simulink model "NMPC_sim"  (R2024b)
settings: Solver=ode4  StartTime=0.0  StopTime=inf  FixedStep=1/60  RelTol=1e-3
values from neighbouring files (symbols this model uses):
  alpha = 2.5    [pre_nmpc_simulink.m]    (also in pre_nmpc_simulink_d10.m = 6.3; pre_nmpc_simulink_d11.m = 7.3; pre_nmpc_simulink_d12.m = 5.8; pre_nmpc_simulink_d13.m = 5.8)
  d = 0.5    [NMPC_System.m]    (also in pre_nmpc_simulink.m = 0.393; pre_nmpc_simulink_d10.m = 0.393; pre_nmpc_simulink_d11.m = 0.393; pre_nmpc_simulink_d12.m = 0.393)
  eta = 0.7    [pre_nmpc_simulink.m]    (also in pre_nmpc_simulink_d10.m = 1.9; pre_nmpc_simulink_d11.m = 1.9; pre_nmpc_simulink_d12.m = 1.4; pre_nmpc_simulink_d13.m = 1.5)
  N = 20    [NMPC_System.m]    (also in pre_nmpc_simulink.m; pre_nmpc_simulink_d10.m; pre_nmpc_simulink_d11.m; pre_nmpc_simulink_d12.m)
  Q_cost = diag([1, 1, 0.1])    [NMPC_System.m]    (also in pre_nmpc_simulink.m = diag([100, 100, 10]); pre_nmpc_simulink_d10.m = diag([100, 100, 10]); pre_nmpc_simulink_d11.m = diag([100, 100, 10]); pre_nmpc_simulink_d12.m = diag([100, 100, 10]))
  r = 0.1    [NMPC_System.m]    (also in pre_nmpc_simulink.m = 0.04445; pre_nmpc_simulink_d10.m = 0.04445; pre_nmpc_simulink_d11.m = 0.04445; pre_nmpc_simulink_d12.m = 0.04445)
  R_cost = diag([0.01, 0.01])    [NMPC_System.m]    (also in pre_nmpc_simulink.m = diag([0.2, 0.1]); pre_nmpc_simulink_d10.m = diag([1.7, 0.1]); pre_nmpc_simulink_d11.m = diag([1.7, 0.1]); pre_nmpc_simulink_d12.m = diag([1.7, 0.1]))
  ts = 0.1    [NMPC_System.m]    (also in pre_nmpc_simulink.m = 0.0166666666667; pre_nmpc_simulink_d10.m = 0.0166666666667; pre_nmpc_simulink_d11.m = 0.0166666666667; pre_nmpc_simulink_d12.m = 0.0166666666667)
  wrwlmax = 10.0    (= 10)    [pre_nmpc_simulink.m]    (also in pre_nmpc_simulink_d10.m; pre_nmpc_simulink_d11.m; pre_nmpc_simulink_d12.m; pre_nmpc_simulink_d13.m)
libraries: simulink x4, quarc_library x3
settings Model: PacingRate=0.032000  Creator=umroot  LastModifiedBy=umroot

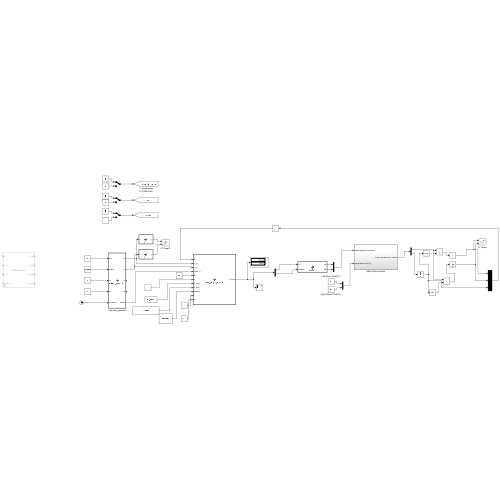
[thumbnail: Simulink's stored preview of the top-level diagram]
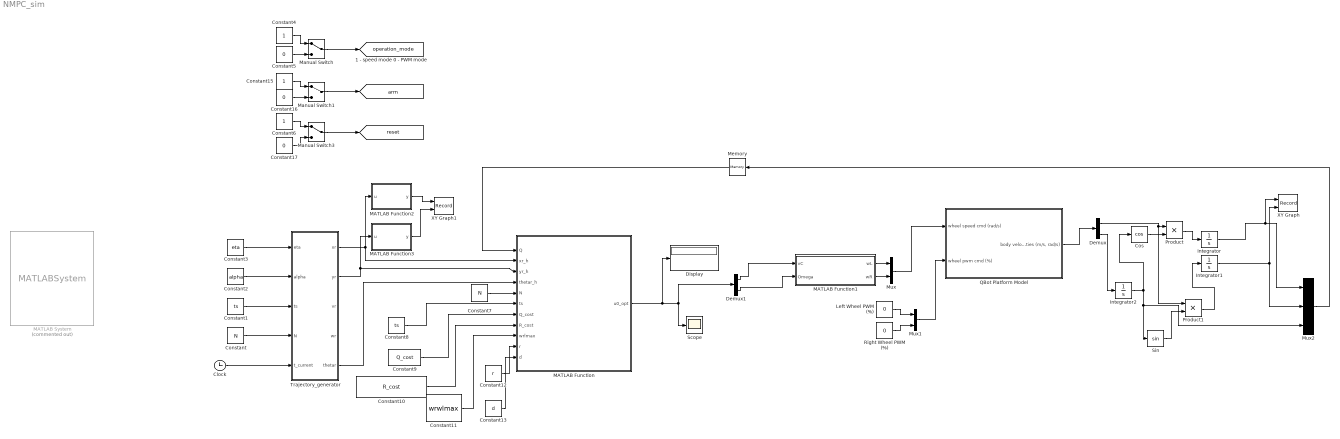
== system NMPC_sim ==
  Clock : Clock
  Constant : Constant  Value=N
  Constant1 : Constant  Value=ts
  Constant10 : Constant  Value=R_cost
  Constant11 : Constant  Value=wrwlmax
  Constant12 : Constant  Value=r
  Constant13 : Constant  Value=d
  Constant15 : Constant
  Constant16 : Constant  Value=0
  Constant17 : Constant  Value=0
  Constant2 : Constant  Value=alpha
  Constant3 : Constant  Value=eta
  Constant4 : Constant
  Constant5 : Constant  Value=0
  Constant6 : Constant
  Constant7 : Constant  Value=N
  Constant8 : Constant  Value=ts
  Constant9 : Constant  Value=Q_cost
  Cos : Trigonometry  Operator=cos
  Demux : Demux  Outputs=2
  Demux1 : Demux  Outputs=2
  Display : Display
  Integrator : Integrator
  Integrator1 : Integrator
  Integrator2 : Integrator  InitialCondition=pi/4
  Left Wheel PWM (%) : Constant  Value=0
  MATLAB Function : MATLAB Function  TreatAsAtomicUnit=on
  MATLAB Function1 : MATLAB Function  TreatAsAtomicUnit=on
  MATLAB Function2 : MATLAB Function  TreatAsAtomicUnit=on
  MATLAB Function3 : MATLAB Function  TreatAsAtomicUnit=on
  MATLAB System : MATLABSystem  Commented=on  System=NMPC_System  N=30  ts=ts  Q_cost=Q_cost  R_cost=R_cost  wrlmax=wrwlmax  r=r  d=d  SimulateUsing=Interpreted execution
      mask Type: NMPC_System
      mask Display:
      | disp('NMPC_System');
      | port_label('input',1,'Q');
      | port_label('input',2,'xr_h');
      | port_label('input',3,'yr_h');
      | port_label('input',4,'thetar_h');
      | port_label('output',1,'x_opt');
      | port_label('output',2,'u_opt');
      | port_label('output',3,'wl_opt');
      | port_label('output',4,'wr_opt');
  Manual Switch : ManualSwitch
  Manual Switch1 : ManualSwitch
  Manual Switch3 : ManualSwitch
  Memory : Memory  InitialCondition=[0;0;pi/4]
  Mux : Mux  Inputs=2
  Mux1 : Mux  Inputs=2
  Mux2 : Mux  Inputs=3
  Product : Product
  Product1 : Product
  QBot Platform Model : Subsystem
  Right Wheel PWM (%) : Constant  Value=0
  Scope : Scope
  Sin : Trigonometry
  Trajectory_generator : MATLAB Function  TreatAsAtomicUnit=on
  XY Graph : Record  FileSettingsInternal="{\"entries\":[{\"content\":{\"excelSettings\":{\"content\":{},\"type\":\"Streamout.ExcelSettings\"}},\"type\":\"Streamout.FileSettingStorage\",\"uuid\":\"\"}],\"packageUris\":[\"http:\\/\\/schema.mathworks.com\\/mf0\\/streamout_blocks\\/R2020a\"],\"version\":\"1.0\"}"  Layout=[1 1]  SignalsInternal="{\"entries\":[{\"content\":{\"signals\":[{\"content\":{\"blockPath\":[],\"dimensions\":[1],\"domain\":\"\",\"lineColor\":\"#a2142f\",\"plots\":[ 1 ],\"port\":1,\"sid\":[\"\"],\"signalID\":1,\"signalName\":\"Integrator\"},\"type\":\"RecordBlkView.Signal\",\"uuid\":\"\"},{\"content\":{\"blockPath\":[],\"dimensions\":[1],\"domain\":\"\",\"lineColor\":\"#139fff\",\"plots\":[ 1 ],\"port\":2,\"sid\":[\"\"],\"signalID\":2,\"signalName\":\"Integrator1\"},\"type\":\"RecordBlkView.Signal\",\"uuid\":\"\"}]},\"type\":\"RecordBlkView.InputSignals\",\"uuid\":\"\"}],\"packageUris\":[\"http:\\/\\/schema.mathworks.com\\/mf0\\/streamout_blocks\\/R2020a\"],\"version\":\"1.0\"}"  VisualizationBindings="{\"xyplotplugin\":{\"info\":[{\"series\":[{\"bindingParametersList\":[{\"parameter\":\"X-Axis\",\"signalID\":1,\"signalName\":\"Integrator\"},{\"parameter\":\"Y-Axis\",\"signalID\":2,\"signalName\":\"Integrator1\"}],\"seriesID\":0}],\"subplotID\":1}]}}"  CompatibilityTag=XY
  XY Graph1 : Record  FileSettingsInternal="{\"entries\":[{\"content\":{\"excelSettings\":{\"content\":{},\"type\":\"Streamout.ExcelSettings\"}},\"type\":\"Streamout.FileSettingStorage\",\"uuid\":\"\"}],\"packageUris\":[\"http:\\/\\/schema.mathworks.com\\/mf0\\/streamout_blocks\\/R2020a\"],\"version\":\"1.0\"}"  Layout=[1 1]  SignalsInternal="{\"entries\":[{\"content\":{\"signals\":[{\"content\":{\"blockPath\":[],\"dimensions\":[1],\"domain\":\"\",\"lineColor\":\"#a2142f\",\"plots\":[ 1 ],\"port\":1,\"sid\":[\"\"],\"signalID\":1,\"signalName\":\"MATLAB Function2\"},\"type\":\"RecordBlkView.Signal\",\"uuid\":\"\"},{\"content\":{\"blockPath\":[],\"dimensions\":[1],\"domain\":\"\",\"lineColor\":\"#64d413\",\"plots\":[ 1 ],\"port\":2,\"sid\":[\"\"],\"signalID\":2,\"signalName\":\"MATLAB Function3\"},\"type\":\"RecordBlkView.Signal\",\"uuid\":\"\"}]},\"type\":\"RecordBlkView.InputSignals\",\"uuid\":\"\"}],\"packageUris\":[\"http:\\/\\/schema.mathworks.com\\/mf0\\/streamout_blocks\\/R2020a\"],\"version\":\"1.0\"}"  VisualizationBindings="{\"xyplotplugin\":{\"info\":[{\"series\":[{\"bindingParametersList\":[{\"parameter\":\"X-Axis\",\"signalID\":1,\"signalName\":\"MATLAB Function2\"},{\"parameter\":\"Y-Axis\",\"signalID\":2,\"signalName\":\"MATLAB Function3\"}],\"seriesID\":0}],\"subplotID\":1}]}}"  CompatibilityTag=XY
  tag scope: arm=global, operation_mode=global, reset=global
  wires:
  Constant/1 -> Trajectory_generator/4(N)
  Constant1/1 -> Trajectory_generator/3(ts)
  Constant2/1 -> Trajectory_generator/2(alpha)
  Constant3/1 -> Trajectory_generator/1(eta)
  Constant7/1 -> MATLAB Function/5(N)
  Constant8/1 -> MATLAB Function/6(ts)
  Constant9/1 -> MATLAB Function/7(Q_cost)
  Constant10/1 -> MATLAB Function/8(R_cost)
  Constant11/1 -> MATLAB Function/9(wrlmax)
  Constant12/1 -> MATLAB Function/10(r)
  Constant13/1 -> MATLAB Function/11(d)
  Trajectory_generator/1(xr) -> MATLAB Function/2(xr_h), MATLAB Function2/1(u)
  Trajectory_generator/2(yr) -> MATLAB Function/3(yr_h), MATLAB Function3/1(u)
  Trajectory_generator/5(thetar) -> MATLAB Function/4(thetar_h)
  MATLAB Function/1(u0_opt) -> Display/1, Demux1/1, Scope/1
  Constant16/1 -> Manual Switch1/2
  Mux1/1 -> QBot Platform Model/2(wheel pwm cmd (%))
  Mux/1 -> QBot Platform Model/1(wheel speed cmd (rad/s))
  Manual Switch1/1 -> [arm]
  Constant6/1 -> Manual Switch3/1
  Constant17/1 -> Manual Switch3/2
  Demux1/2 -> MATLAB Function1/2(Omega)
  Constant5/1 -> Manual Switch/2
  Constant4/1 -> Manual Switch/1
  Right Wheel PWM (%)/1 -> Mux1/2
  Manual Switch3/1 -> [reset]
  Manual Switch/1 -> [operation_mode]
  Left Wheel PWM (%)/1 -> Mux1/1
  MATLAB Function1/1(wL) -> Mux/1
  Demux1/1 -> MATLAB Function1/1(vC)
  MATLAB Function1/2(wR) -> Mux/2
  Constant15/1 -> Manual Switch1/1
  Integrator/1 -> Mux2/1, XY Graph/1
  Integrator1/1 -> Mux2/2, XY Graph/2
  Demux/2 -> Integrator2/1
  Integrator2/1 -> Cos/1, Mux2/3, Sin/1
  Cos/1 -> Product/2
  Demux/1 -> Product1/1, Product/1
  Product/1 -> Integrator/1
  Sin/1 -> Product1/2
  Product1/1 -> Integrator1/1
  Mux2/1 -> Memory/1
  Memory/1 -> MATLAB Function/1(Q)
  Clock/1 -> Trajectory_generator/5(t_current)
  QBot Platform Model/1("body velocities (m/s, rad/s)") -> Demux/1
  MATLAB Function2/1(y) -> XY Graph1/1
  MATLAB Function3/1(y) -> XY Graph1/2

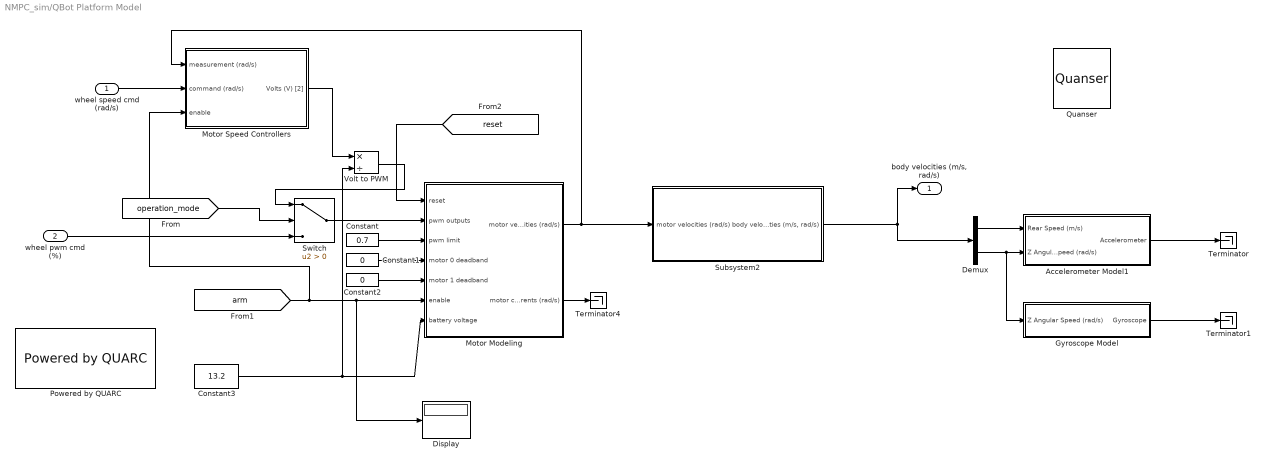
== system NMPC_sim/QBot Platform Model ==
  wheel speed cmd (rad/s) : Inport
  wheel pwm cmd (%) : Inport  Port=2
  Accelerometer Model1 : Subsystem
  Constant : Constant  Value=0.7
  Constant1 : Constant  Value=0
  Constant2 : Constant  Value=0
  Constant3 : Constant  Value=13.2
  Demux : Demux  Outputs=2
  Display : Display
  Gyroscope Model : Subsystem
  Motor Modeling : Subsystem
  Motor Speed Controllers : Subsystem
  Powered by QUARC : quarc_library/Logos/Powered by QUARC
  Quanser : quarc_library/Logos/Quanser
  Subsystem2 : Subsystem
  Switch : Switch  Criteria=u2 > Threshold  SaturateOnIntegerOverflow=off  InputSameDT=off
  Terminator : Terminator
  Terminator1 : Terminator
  Terminator4 : Terminator
  Volt to PWM : Product  Inputs=*/
  "body velocities (m/s, rad/s)" : Outport
  wires:
  [operation_mode] -> Switch/2
  Constant/1 -> Motor Modeling/3(pwm limit)
  Motor Speed Controllers/1(Volts (V) [2]) -> Volt to PWM/1
  Switch/1 -> Motor Modeling/2(pwm outputs)
  Constant1/1 -> Motor Modeling/4(motor 0 deadband)
  [reset] -> Motor Modeling/1(reset)
  wheel speed cmd (rad/s)/1 -> Motor Speed Controllers/2(command (rad/s))
  Constant2/1 -> Motor Modeling/5(motor 1 deadband)
  Constant3/1 -> Motor Modeling/7(battery voltage), Volt to PWM/2
  [arm] -> Motor Modeling/6(enable), Display/1, Motor Speed Controllers/3(enable)
  Volt to PWM/1 -> Switch/1
  wheel pwm cmd (%)/1 -> Switch/3
  Motor Modeling/1(motor velocities (rad/s)) -> Subsystem2/1("motor velocities (rad/s) "), Motor Speed Controllers/1(measurement (rad/s))
  Demux/1 -> Accelerometer Model1/1(Rear Speed (m/s))
  Demux/2 -> Gyroscope Model/1(Z Angular Speed (rad/s)), Accelerometer Model1/2(Z Angular Speed (rad/s))
  Subsystem2/1("body velocities (m/s, rad/s)") -> "body velocities (m/s, rad/s)"/1, Demux/1
  Gyroscope Model/1(Gyroscope) -> Terminator1/1
  Accelerometer Model1/1(Accelerometer) -> Terminator/1
  Motor Modeling/2(motor currents (rad/s)) -> Terminator4/1

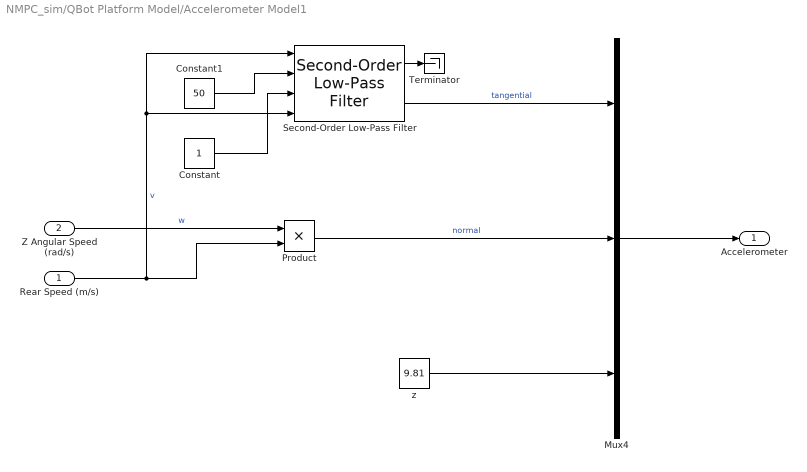
== system NMPC_sim/QBot Platform Model/Accelerometer Model1 ==
  Rear Speed (m/s) : Inport
  Z Angular Speed (rad/s) : Inport  Port=2
  Constant : Constant
  Constant1 : Constant  Value=50
  Mux4 : Mux  Inputs=3
  Product : Product
  Second-Order Low-Pass Filter : quarc_library/Continuous/Second-Order Low-Pass Filter  params_source=External (input ports)  input_width=1  input_zeta=1  input_init=0
  Terminator : Terminator
  z : Constant  Value=9.81
  Accelerometer : Outport
  wires:
  Z Angular Speed (rad/s)/1 -> Product/1  "w"
  Second-Order Low-Pass Filter/2 -> Mux4/1  "tangential"
  Rear Speed (m/s)/1 -> Second-Order Low-Pass Filter/4, Second-Order Low-Pass Filter/1, Product/2  "v"
  Product/1 -> Mux4/2  "normal"
  Mux4/1 -> Accelerometer/1
  z/1 -> Mux4/3
  Second-Order Low-Pass Filter/1 -> Terminator/1
  Constant/1 -> Second-Order Low-Pass Filter/3
  Constant1/1 -> Second-Order Low-Pass Filter/2

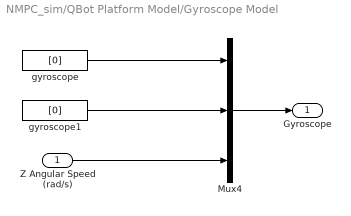
== system NMPC_sim/QBot Platform Model/Gyroscope Model ==
  Z Angular Speed (rad/s) : Inport
  Mux4 : Mux  Inputs=3
  gyroscope : Constant  Value=[0]
  gyroscope1 : Constant  Value=[0]
  Gyroscope : Outport
  wires:
  Z Angular Speed (rad/s)/1 -> Mux4/3
  Mux4/1 -> Gyroscope/1
  gyroscope/1 -> Mux4/1
  gyroscope1/1 -> Mux4/2

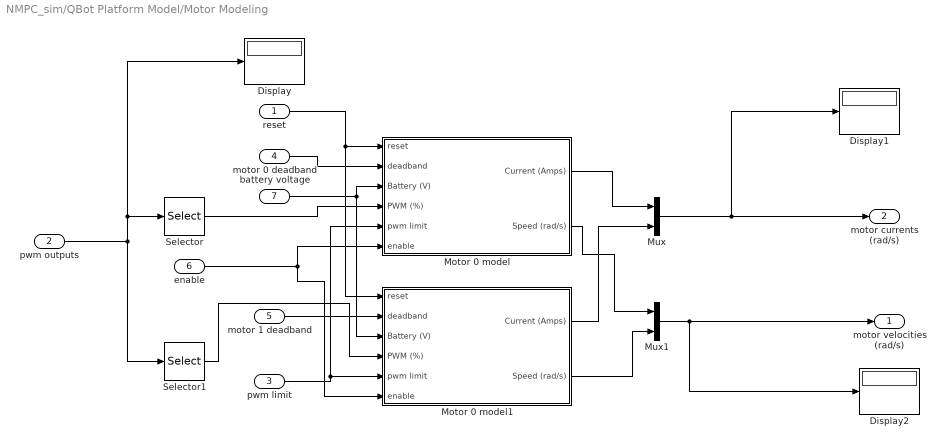
== system NMPC_sim/QBot Platform Model/Motor Modeling ==
  reset : Inport
  pwm outputs : Inport  Port=2
  pwm limit : Inport  Port=3
  motor 0 deadband : Inport  Port=4
  motor 1 deadband : Inport  Port=5
  enable : Inport  Port=6
  battery voltage : Inport  Port=7
  Display : Display
  Display1 : Display
  Display2 : Display
  Motor 0 model : Subsystem
  Motor 0 model1 : Subsystem
  Mux : Mux  Inputs=2
  Mux1 : Mux  Inputs=2
  Selector : Selector  InputPortWidth=2  IndexOptions=Index vector (dialog)  Indices=1  OutputSizes=1
  Selector1 : Selector  InputPortWidth=2  IndexOptions=Index vector (dialog)  Indices=2  OutputSizes=1
  motor velocities (rad/s) : Outport
  motor currents (rad/s) : Outport  Port=2
  wires:
  reset/1 -> Motor 0 model1/1(reset), Motor 0 model/1(reset)
  Motor 0 model1/1(Current (Amps)) -> Mux/2
  battery voltage/1 -> Motor 0 model1/3(Battery (V)), Motor 0 model/3(Battery (V))
  Motor 0 model/1(Current (Amps)) -> Mux/1
  Motor 0 model1/2(Speed (rad/s)) -> Mux1/2
  Motor 0 model/2(Speed (rad/s)) -> Mux1/1
  Mux/1 -> motor currents (rad/s)/1, Display1/1
  Mux1/1 -> motor velocities (rad/s)/1, Display2/1
  pwm outputs/1 -> Display/1, Selector/1, Selector1/1
  motor 0 deadband/1 -> Motor 0 model/2(deadband)
  motor 1 deadband/1 -> Motor 0 model1/2(deadband)
  Selector/1 -> Motor 0 model/4(PWM (%))
  Selector1/1 -> Motor 0 model1/4(PWM (%))
  pwm limit/1 -> Motor 0 model1/5(pwm limit), Motor 0 model/5(pwm limit)
  enable/1 -> Motor 0 model/6(enable), Motor 0 model1/6(enable)

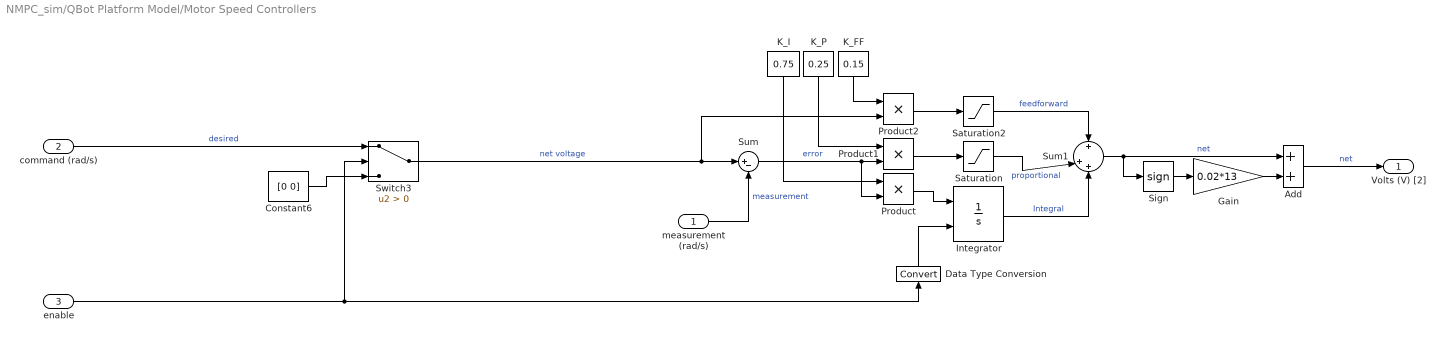
== system NMPC_sim/QBot Platform Model/Motor Speed Controllers ==
  measurement (rad/s) : Inport
  command (rad/s) : Inport  Port=2
  enable : Inport  Port=3
  Add : Sum
  Constant6 : Constant  Value=[0 0]
  Data Type Conversion : DataTypeConversion  SaturateOnIntegerOverflow=off  RndMeth=Floor
  Gain : Gain  Gain=0.02*13
  Integrator : Integrator  ExternalReset=either  InitialCondition=[0 0]  LimitOutput=on  UpperSaturationLimit=[2 2]  LowerSaturationLimit=[-2 -2]
  K_FF : Constant  Value=0.15
  K_I : Constant  Value=0.75
  K_P : Constant  Value=0.25
  Product : Product
  Product1 : Product
  Product2 : Product
  Saturation : Saturate  UpperLimit=[5 5]  LowerLimit=[-5 -5]
  Saturation2 : Saturate  UpperLimit=[5 5]  LowerLimit=[-5 -5]
  Sign : Signum
  Sum : Sum  Inputs=|+-
  Sum1 : Sum  Inputs=+|++
  Switch3 : Switch  Criteria=u2 > Threshold  SaturateOnIntegerOverflow=off  InputSameDT=off
  Volts (V) [2] : Outport
  wires:
  Product1/1 -> Saturation/1
  Product/1 -> Integrator/1
  Sum/1 -> Product/2, Product1/2  "error"
  measurement (rad/s)/1 -> Sum/2  "measurement"
  command (rad/s)/1 -> Switch3/1  "desired"
  Data Type Conversion/1 -> Integrator/2
  Add/1 -> Volts (V) [2]/1  "net"
  enable/1 -> Switch3/2, Data Type Conversion/1
  Product2/1 -> Saturation2/1
  Constant6/1 -> Switch3/3
  Switch3/1 -> Product2/2, Sum/1  "net voltage"
  K_I/1 -> Product/1
  K_P/1 -> Product1/1
  K_FF/1 -> Product2/1
  Saturation/1 -> Sum1/2  "proportional"
  Saturation2/1 -> Sum1/1  "feedforward"
  Sum1/1 -> Sign/1, Add/1  "net"
  Sign/1 -> Gain/1
  Gain/1 -> Add/2
  Integrator/1 -> Sum1/3  "Integral"

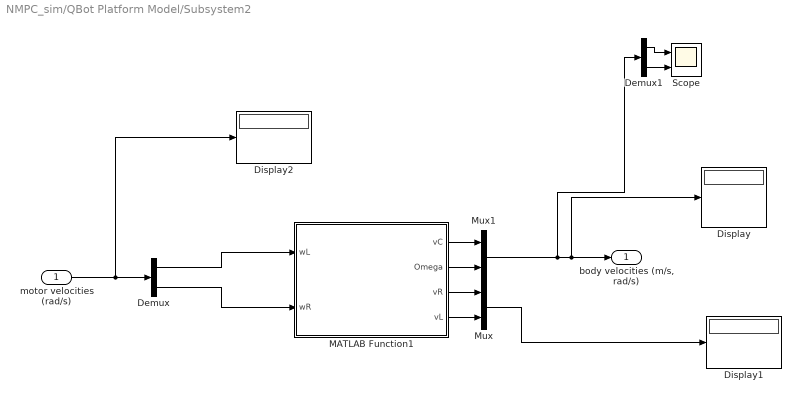
== system NMPC_sim/QBot Platform Model/Subsystem2 ==
  "motor velocities (rad/s) " : Inport
  Demux : Demux  Outputs=2
  Demux1 : Demux  Outputs=2
  Display : Display
  Display1 : Display
  Display2 : Display
  MATLAB Function1 : MATLAB Function  TreatAsAtomicUnit=on
  Mux : Mux  Inputs=2
  Mux1 : Mux  Inputs=2
  Scope : Scope  NumInputPorts=2
  "body velocities (m/s, rad/s)" : Outport
  wires:
  MATLAB Function1/2(Omega) -> Mux1/2
  MATLAB Function1/1(vC) -> Mux1/1
  MATLAB Function1/4(vL) -> Mux/2
  MATLAB Function1/3(vR) -> Mux/1
  Mux1/1 -> Demux1/1, Display/1, "body velocities (m/s, rad/s)"/1
  Mux/1 -> Display1/1
  "motor velocities (rad/s) "/1 -> Display2/1, Demux/1
  Demux/1 -> MATLAB Function1/1(wL)
  Demux/2 -> MATLAB Function1/2(wR)
  Demux1/2 -> Scope/2
  Demux1/1 -> Scope/1

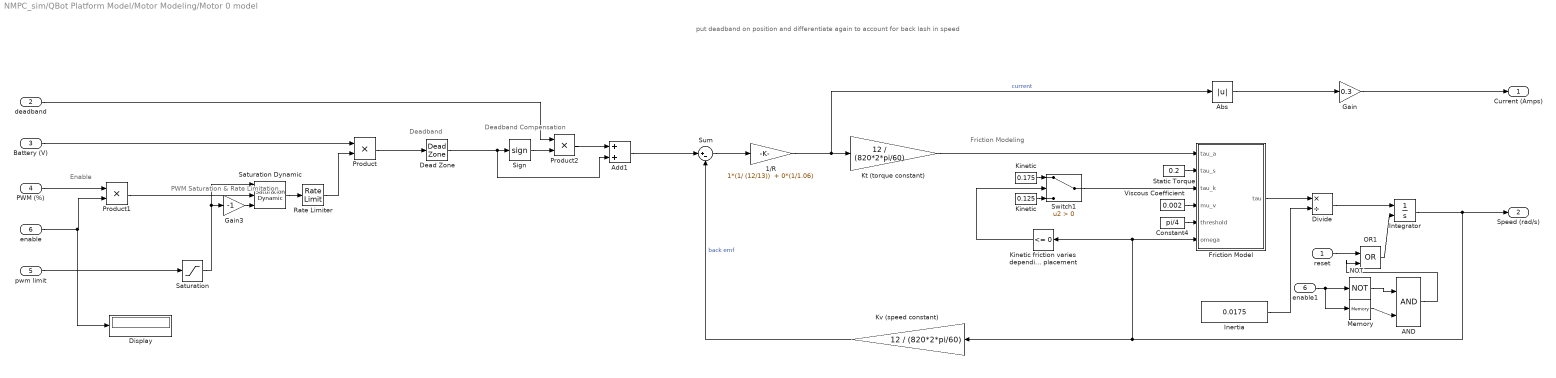
== system NMPC_sim/QBot Platform Model/Motor Modeling/Motor 0 model ==
  note: Friction Modeling
  note: Deadband
  note: Deadband Compensation
  note: PWM Saturation & Rate Limitation
  note: Enable
  note: put deadband on position and differentiate again to account for back lash in speed
  reset : Inport
  deadband : Inport  Port=2
  Battery (V) : Inport  Port=3
  PWM (%) : Inport  Port=4
  pwm limit : Inport  Port=5
  enable : Inport  Port=6
  1/R : Gain  Gain="1*(1/ (12/13))  + 0*(1/1.06)"
  AND : Logic  IconShape=distinctive  AllPortsSameDT=off  OutDataTypeStr=boolean
  Abs : Abs  SaturateOnIntegerOverflow=off
  Add1 : Sum
  Constant4 : Constant  Value=pi/4
  Dead Zone : DeadZone  LowerValue=-0.2  UpperValue=0.2
  Display : Display
  Divide : Product  Inputs=*/
  Friction Model : MATLAB Function  TreatAsAtomicUnit=on
  Gain : Gain  Gain=0.3
  Gain3 : Gain  Gain=-1
  Inertia : Constant  Value=0.0175
  Integrator : Integrator  ExternalReset=rising
  Kinetic : Constant  Value=0.125
  "Kinetic  " : Constant  Value=0.175
  "Kinetic friction varies depending on motor direction due to non symmetric front-back CG placement " : simulink/Logic and Bit Operations/Compare To Constant  relop=<=  const=0  OutDataTypeStr=boolean
  Kt (torque constant) : Gain  Gain=12 / (820*2*pi/60)
  Kv (speed constant) : Gain  Gain=12 / (820*2*pi/60)
  Memory : Memory  InheritSampleTime=on
  NOT : Logic  Operator=NOT  IconShape=distinctive  AllPortsSameDT=off  OutDataTypeStr=boolean
  OR1 : Logic  Operator=OR  IconShape=distinctive  AllPortsSameDT=off  OutDataTypeStr=boolean
  Product : Product
  Product1 : Product
  Product2 : Product
  Rate Limiter : RateLimiter  RisingSlewLimit=2.75  FallingSlewLimit=-2.75  SampleTimeMode=inherited
  Saturation : Saturate  UpperLimit=0.7  LowerLimit=0
  Saturation Dynamic : simulink/Discontinuities/Saturation Dynamic  OutMin=[]  OutMax=[]  OutDataTypeStr=Inherit: Same as second input  OutDataType=fixdt(1, 16)  OutScaling=2^-10  DoSatur=off
  Sign : Signum
  Static Torque : Constant  Value=0.2
  Sum : Sum  Inputs=|+-
  Switch1 : Switch  Criteria=u2 > Threshold  SaturateOnIntegerOverflow=off  InputSameDT=off
  Viscous Coefficient : Constant  Value=0.002
  enable1 : InportShadow  Port=6
  Current (Amps) : Outport
  Speed (rad/s) : Outport  Port=2
  wires:
  Static Torque/1 -> Friction Model/2(tau_s)
  Switch1/1 -> Friction Model/3(tau_k)
  Constant4/1 -> Friction Model/5(threshold)
  Integrator/1 -> Speed (rad/s)/1, "Kinetic friction varies depending on motor direction due to non symmetric front-back CG placement "/1, Friction Model/6(omega), Kv (speed constant)/1
  Kv (speed constant)/1 -> Sum/2  "back emf"
  Add1/1 -> Sum/1
  Sign/1 -> Product2/2
  Divide/1 -> Integrator/1
  Sum/1 -> 1/R/1
  Friction Model/1(tau) -> Divide/1
  Kt (torque constant)/1 -> Friction Model/1(tau_a)
  Dead Zone/1 -> Add1/2, Sign/1
  Battery (V)/1 -> Product/1
  Product1/1 -> Saturation Dynamic/2
  Abs/1 -> Gain/1
  reset/1 -> OR1/1
  Product/1 -> Dead Zone/1
  Rate Limiter/1 -> Product/2
  Saturation Dynamic/1 -> Rate Limiter/1
  1/R/1 -> Abs/1, Kt (torque constant)/1  "current"
  Inertia/1 -> Divide/2
  "Kinetic  "/1 -> Switch1/1
  Kinetic/1 -> Switch1/3
  Viscous Coefficient/1 -> Friction Model/4(mu_v)
  "Kinetic friction varies depending on motor direction due to non symmetric front-back CG placement "/1 -> Switch1/2
  pwm limit/1 -> Saturation/1
  Saturation/1 -> Gain3/1, Saturation Dynamic/1
  Gain3/1 -> Saturation Dynamic/3
  enable/1 -> Display/1, Product1/2
  PWM (%)/1 -> Product1/1
  Product2/1 -> Add1/1
  deadband/1 -> Product2/1
  Gain/1 -> Current (Amps)/1
  enable1/1 -> Memory/1, NOT/1
  OR1/1 -> Integrator/2
  Memory/1 -> AND/2
  NOT/1 -> AND/1
  AND/1 -> OR1/2

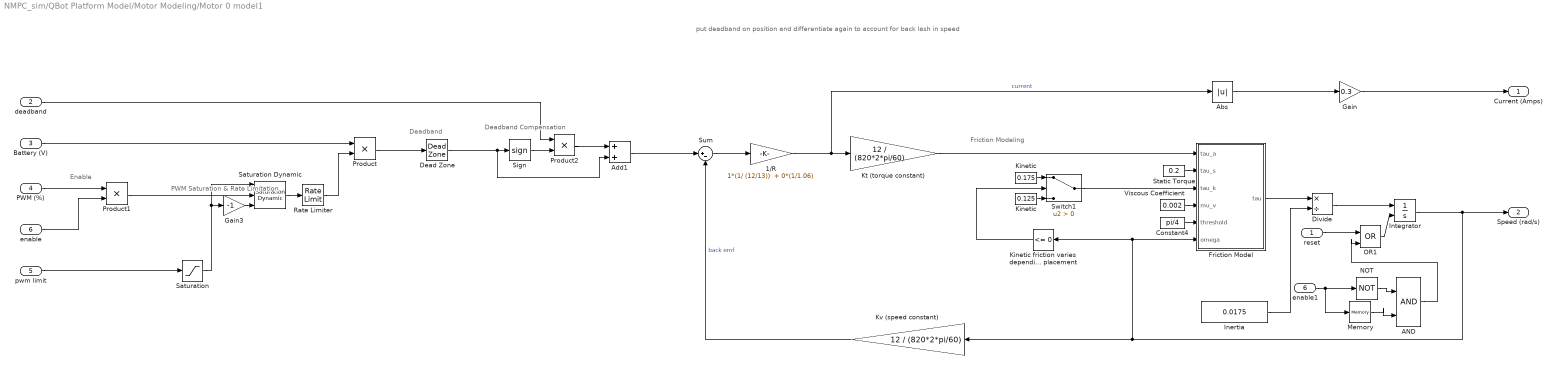
== system NMPC_sim/QBot Platform Model/Motor Modeling/Motor 0 model1 ==
  note: put deadband on position and differentiate again to account for back lash in speed
  note: Enable
  note: PWM Saturation & Rate Limitation
  note: Deadband Compensation
  note: Deadband
  note: Friction Modeling
  reset : Inport
  deadband : Inport  Port=2
  Battery (V) : Inport  Port=3
  PWM (%) : Inport  Port=4
  pwm limit : Inport  Port=5
  enable : Inport  Port=6
  1/R : Gain  Gain="1*(1/ (12/13))  + 0*(1/1.06)"
  AND : Logic  IconShape=distinctive  AllPortsSameDT=off  OutDataTypeStr=boolean
  Abs : Abs  SaturateOnIntegerOverflow=off
  Add1 : Sum
  Constant4 : Constant  Value=pi/4
  Dead Zone : DeadZone  LowerValue=-0.2  UpperValue=0.2
  Divide : Product  Inputs=*/
  Friction Model : MATLAB Function  TreatAsAtomicUnit=on
  Gain : Gain  Gain=0.3
  Gain3 : Gain  Gain=-1
  Inertia : Constant  Value=0.0175
  Integrator : Integrator  ExternalReset=rising
  Kinetic : Constant  Value=0.125
  "Kinetic  " : Constant  Value=0.175
  "Kinetic friction varies depending on motor direction due to non symmetric front-back CG placement " : simulink/Logic and Bit Operations/Compare To Constant  relop=<=  const=0  OutDataTypeStr=boolean
  Kt (torque constant) : Gain  Gain=12 / (820*2*pi/60)
  Kv (speed constant) : Gain  Gain=12 / (820*2*pi/60)
  Memory : Memory  InheritSampleTime=on
  NOT : Logic  Operator=NOT  IconShape=distinctive  AllPortsSameDT=off  OutDataTypeStr=boolean
  OR1 : Logic  Operator=OR  IconShape=distinctive  AllPortsSameDT=off  OutDataTypeStr=boolean
  Product : Product
  Product1 : Product
  Product2 : Product
  Rate Limiter : RateLimiter  RisingSlewLimit=2.75  FallingSlewLimit=-2.75  SampleTimeMode=inherited
  Saturation : Saturate  UpperLimit=0.7  LowerLimit=0
  Saturation Dynamic : simulink/Discontinuities/Saturation Dynamic  OutMin=[]  OutMax=[]  OutDataTypeStr=Inherit: Same as second input  OutDataType=fixdt(1, 16)  OutScaling=2^-10  DoSatur=off
  Sign : Signum
  Static Torque : Constant  Value=0.2
  Sum : Sum  Inputs=|+-
  Switch1 : Switch  Criteria=u2 > Threshold  SaturateOnIntegerOverflow=off  InputSameDT=off
  Viscous Coefficient : Constant  Value=0.002
  enable1 : InportShadow  Port=6
  Current (Amps) : Outport
  Speed (rad/s) : Outport  Port=2
  wires:
  NOT/1 -> AND/1
  Memory/1 -> AND/2
  OR1/1 -> Integrator/2
  enable1/1 -> Memory/1, NOT/1
  Gain/1 -> Current (Amps)/1
  deadband/1 -> Product2/1
  Product2/1 -> Add1/1
  PWM (%)/1 -> Product1/1
  enable/1 -> Product1/2
  Gain3/1 -> Saturation Dynamic/3
  Saturation/1 -> Saturation Dynamic/1, Gain3/1
  pwm limit/1 -> Saturation/1
  "Kinetic friction varies depending on motor direction due to non symmetric front-back CG placement "/1 -> Switch1/2
  Viscous Coefficient/1 -> Friction Model/4(mu_v)
  Kinetic/1 -> Switch1/3
  "Kinetic  "/1 -> Switch1/1
  Inertia/1 -> Divide/2
  1/R/1 -> Kt (torque constant)/1, Abs/1  "current"
  Saturation Dynamic/1 -> Rate Limiter/1
  Rate Limiter/1 -> Product/2
  Product/1 -> Dead Zone/1
  reset/1 -> OR1/1
  Abs/1 -> Gain/1
  Product1/1 -> Saturation Dynamic/2
  Battery (V)/1 -> Product/1
  Dead Zone/1 -> Sign/1, Add1/2
  Kt (torque constant)/1 -> Friction Model/1(tau_a)
  Friction Model/1(tau) -> Divide/1
  Sum/1 -> 1/R/1
  Divide/1 -> Integrator/1
  Sign/1 -> Product2/2
  Add1/1 -> Sum/1
  Kv (speed constant)/1 -> Sum/2  "back emf"
  Integrator/1 -> Kv (speed constant)/1, Friction Model/6(omega), "Kinetic friction varies depending on motor direction due to non symmetric front-back CG placement "/1, Speed (rad/s)/1
  Constant4/1 -> Friction Model/5(threshold)
  Switch1/1 -> Friction Model/3(tau_k)
  Static Torque/1 -> Friction Model/2(tau_s)
  AND/1 -> OR1/2

== matlab function NMPC_sim/MATLAB Function ==
  data: Q input; xr_h input; yr_h input; thetar_h input; N input; ts input; Q_cost input; R_cost input; wrlmax input; r input; d input; u0_opt output size=[2,1]
function u0_opt = solve_nmpc_fmincon(Q, xr_h, yr_h, thetar_h, N, ts, Q_cost, R_cost, wrlmax, r, d)
    % NMPC solver using fmincon with fixed-size output for Simulink compatibility
    
    % Define state and control dimensions
    nx = 3;  % [x, y, theta]
    nu = 2;  % [v, omega]

    % Fixed-size output initialization
    u0_opt = NaN(nu, 1);

    % Lower and upper bounds for control inputs
    v_min = -r * wrlmax;
    v_max = r * wrlmax;
    omega_min = -r * wrlmax / d;
    omega_max = r * wrlmax / d;

    lb = [repmat(-inf, nx*(N+1), 1); repmat([v_min; omega_min], N, 1)];
    ub = [repmat(inf, nx*(N+1), 1); repmat([v_max; omega_max], N, 1)];

    % Initial guess for states and controls
    x_init = repmat(Q, 1, N+1);
    u_init = zeros(nu, N);
    x_u_init = [x_init(:); u_init(:)];  % Flatten initial values

    % Objective function
    objective = @(x_u) compute_objective(x_u, N, ts, Q_cost, R_cost, xr_h, yr_h, thetar_h, nx, nu, r, d);

    % Constraints function
    constraints = @(x_u) compute_constraints(x_u, N, ts, Q, nx, nu, r, d);

    % Solver options
    options = optimoptions('fmincon', 'Display', 'off', 'Algorithm', 'sqp');
    options.MaxIterations = 100;
    options.ConstraintTolerance = 1.0e-6;
    options.OptimalityTolerance = 1.0e-2;

    % Solve using fmincon

    [x_u_opt, ~] = fmincon(objective, x_u_init, [], [], [], [], lb, ub, constraints, options);
    
    % Extract optimal control input for the first step
    u_opt = reshape(x_u_opt(nx*(N+1)+1:end), nu, N);
    u0_opt = u_opt(:,1);


end


% Compute the objective function
function obj = compute_objective(x_u, N, ts, Q_cost, R_cost, xr_h, yr_h, thetar_h, nx, nu, r, d)
    x = reshape(x_u(1:nx*(N+1)), nx, N+1);
    u = reshape(x_u(nx*(N+1)+1:end), nu, N);

    objective = 0;
    for t = 1:N
        % State tracking error
        state_error = x(:, t) - [xr_h(t); yr_h(t); thetar_h(t)];
        objective = objective + state_error' * Q_cost * state_error + u(:, t)' * R_cost * u(:, t);
    end

    % Terminal cost
    state_error = x(:, N+1) - [xr_h(N+1); yr_h(N+1); thetar_h(N+1)];
    objective = objective + state_error' * Q_cost * state_error;
    obj = objective;
end

% Compute the constraints
function [c, ceq] = compute_constraints(x_u, N, ts, Q, nx, nu, r, d)
    x = reshape(x_u(1:nx*(N+1)), nx, N+1);
    u = reshape(x_u(nx*(N+1)+1:end), nu, N);

    % Initialize constraints
    c = [];  % Inequality constraints (none)
    ceq = [];

    % Initial condition constraint
    ceq = [ceq; x(:, 1) - Q];

    % Dynamic constraints
    for t = 1:N
        % Differential drive model
        x_next = x(:, t) + ts * [
            u(1, t) * cos(x(3, t));
            u(1, t) * sin(x(3, t));
            u(2, t)
        ];

        % Add the dynamics constraint (x_next == x(t+1))
        ceq = [ceq; x(:, t+1) - x_next];

        % Control input constraints are handled in bounds
    end
end

== matlab function NMPC_sim/Trajectory_generator ==
  data: eta input; xr output; alpha input; ts input; N input; t_current input; yr output; vr output; wr output; thetar output
function [xr, yr, vr, wr, thetar] = predict_waypoints(eta, alpha, ts, N, t_current)
%#codegen
    % Define maximum prediction horizon (adjust as needed)
    max_N = 100;  % Set this based on your expected upper limit for N
    N = N+1;
    % Preallocate arrays with a fixed size
    xr = zeros(max_N, 1);
    yr = zeros(max_N, 1);
    vr = zeros(max_N, 1);
    wr = zeros(max_N, 1);
    thetar = zeros(max_N, 1);
    
    % Define time vector for prediction horizon
    k_end = t_current + max_N * ts;
    k = 0:ts:k_end;
    
    % Position trajectory
    x_temp = eta * sin(k / alpha);
    y_temp = eta * sin(k / (2 * alpha));
    
    % Velocity trajectory
    xpr = eta * cos(k / alpha) / alpha;
    ypr = eta * cos(k / (2 * alpha)) / (2 * alpha);
    
    % Acceleration trajectory
    xppr = -eta * sin(k / alpha) / alpha^2;
    yppr = -eta * sin(k / (2 * alpha)) / (2 * alpha)^2;
    
    % Driving velocity reference
    v_temp = sqrt(xpr.^2 + ypr.^2);
    w_temp = (yppr .* xpr - xppr .* ypr) ./ (xpr.^2 + ypr.^2);
    
    % Orientation reference
    theta_temp = atan2(ypr, xpr);
    theta_temp = unwrap(theta_temp);
    
    % Find current index based on time
    k_current_idx = round(t_current / ts) + 1;
    k_future_idx = k_current_idx:k_current_idx + N - 1;
    
    % Ensure indices are within bounds
    k_future_idx(k_future_idx > length(x_temp)) = length(x_temp);
    
    % Assign values to preallocated arrays
    xr(1:N) = x_temp(k_future_idx);
    yr(1:N) = y_temp(k_future_idx);
    vr(1:N) = v_temp(k_future_idx);
    wr(1:N) = w_temp(k_future_idx);
    thetar(1:N) = theta_temp(k_future_idx);
end

== matlab function NMPC_sim/MATLAB Function2 ==
  data: u input; y output
function y = fcn(u)

y = u(1)

== matlab function NMPC_sim/MATLAB Function3 ==
  data: u input; y output
function y = fcn(u)

y = u(1);

== matlab function NMPC_sim/QBot Platform Model/Motor Modeling/Motor 0 model/Friction Model ==
  data: tau_a input; tau output; tau_s input; tau_k input; mu_v input; threshold input; omega input
function tau = fcn(tau_a, tau_s, tau_k, mu_v, threshold, omega)

% Friction Model:
% tau           - output torque
% tau_a         - applied torque
% tau_s         - static friction torque
% tau_k         - kinetic friction torque
% tau_v         - viscous friction torque
% threshold     - threshold under which you want omega to be considered 0
% omega         - angular speed

% v1.0 Murtaza Bohra
not_moving = 0;
if abs(omega) <= threshold
    not_moving = 1;
end

if (abs(tau_a) < tau_s)&&(not_moving)
    tau = 0;
else
    tau = tau_a - tau_k*sign(omega) - mu_v*omega;
end

== matlab function NMPC_sim/MATLAB Function1 ==
  data: wL output; vC input; wR output; Omega input
function [wL, wR] = invKin(vC , Omega)

% wheelbase
d=0.3928; 

% calculate wheel linear velocities
vR = vC + Omega*d/2;
vL = vC - Omega*d/2;

% calculate wheel angular velocities
wheelRadius = 3.5*0.0254/2;

wR = vR/ wheelRadius;
wL = vL/ wheelRadius;

== matlab function NMPC_sim/QBot Platform Model/Motor Modeling/Motor 0 model1/Friction Model ==
  data: tau_a input; tau output; tau_s input; tau_k input; mu_v input; threshold input; omega input
function tau = fcn(tau_a, tau_s, tau_k, mu_v, threshold, omega)

% Friction Model:
% tau           - output torque
% tau_a         - applied torque
% tau_s         - static friction torque
% tau_k         - kinetic friction torque
% tau_v         - viscous friction torque
% threshold     - threshold under which you want omega to be considered 0
% omega         - angular speed

% v1.0 Murtaza Bohra
not_moving = 0;
if abs(omega) <= threshold
    not_moving = 1;
end

if (abs(tau_a) < tau_s)&&(not_moving)
    tau = 0;
else
    tau = tau_a - tau_k*sign(omega) - mu_v*omega;
end

== matlab function NMPC_sim/QBot Platform Model/Subsystem2/MATLAB Function1 ==
  data: vC output; wL input; Omega output; wR input; vR output; vL output
function [vC, Omega, vR, vL] = forKin(wL, wR)

% calculate wheel angular velocities
wheelRadius = 3.5*0.0254/2;

vR = wR * wheelRadius;
vL = wL * wheelRadius;

% wheelbase
d=0.3928; 

% calculate wheel linear velocities
vC = (vR + vL)/2;
Omega = (vR - vL)/d;
